simulink model "Quan"  (R2016a)
settings: Solver=VariableStepAuto  StartTime=0.0  StopTime=5000  FixedStep=0.1  RelTol=1e-3
settings Model: Creator=xin  LastModifiedBy=xin

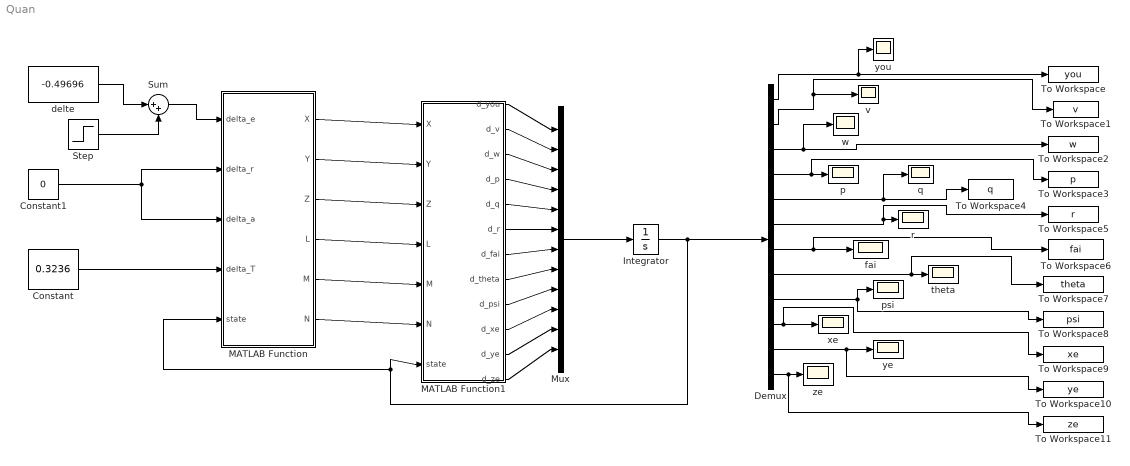
== system Quan ==
  Constant : Constant  Value=0.3236
  Constant1 : Constant  Value=0
  Demux : Demux  Outputs=12
  Integrator : Integrator  InitialCondition=[189.1684 0 17.7568 0 0 0 0 0.0936 0 0 0 0]
  MATLAB Function : MATLAB Function  TreatAsAtomicUnit=on
  MATLAB Function1 : MATLAB Function  TreatAsAtomicUnit=on
  Mux : Mux  Inputs=12
  Step : Step  Time=0  After=0.025  SampleTime=0
  Sum : Sum  Inputs=|++
  To Workspace : ToWorkspace  VariableName=you  SaveFormat=Timeseries  SampleTime=-1
  To Workspace1 : ToWorkspace  VariableName=v  SaveFormat=Timeseries  SampleTime=-1
  To Workspace10 : ToWorkspace  VariableName=ye  SaveFormat=Timeseries  SampleTime=-1
  To Workspace11 : ToWorkspace  VariableName=ze  SaveFormat=Timeseries  SampleTime=-1
  To Workspace2 : ToWorkspace  VariableName=w  SaveFormat=Timeseries  SampleTime=-1
  To Workspace3 : ToWorkspace  VariableName=p  SaveFormat=Timeseries  SampleTime=-1
  To Workspace4 : ToWorkspace  VariableName=q  SaveFormat=Timeseries  SampleTime=-1
  To Workspace5 : ToWorkspace  VariableName=r  SaveFormat=Timeseries  SampleTime=-1
  To Workspace6 : ToWorkspace  VariableName=fai  SaveFormat=Timeseries  SampleTime=-1
  To Workspace7 : ToWorkspace  VariableName=theta  SaveFormat=Timeseries  SampleTime=-1
  To Workspace8 : ToWorkspace  VariableName=psi  SaveFormat=Timeseries  SampleTime=-1
  To Workspace9 : ToWorkspace  VariableName=xe  SaveFormat=Timeseries  SampleTime=-1
  delte : Constant  Value=-0.49696
  fai : Scope
  p : Scope
  psi : Scope
  q : Scope
  r : Scope
  "theta " : Scope
  v : Scope
  w : Scope
  xe : Scope
  ye : Scope
  you : Scope
  "ze " : Scope
  wires:
  MATLAB Function/1(X) -> MATLAB Function1/1(X)
  MATLAB Function/2(Y) -> MATLAB Function1/2(Y)
  MATLAB Function/3(Z) -> MATLAB Function1/3(Z)
  MATLAB Function/4(L) -> MATLAB Function1/4(L)
  MATLAB Function/5(M) -> MATLAB Function1/5(M)
  MATLAB Function/6(N) -> MATLAB Function1/6(N)
  MATLAB Function1/1(d_you) -> Mux/1
  MATLAB Function1/2(d_v) -> Mux/2
  MATLAB Function1/3(d_w) -> Mux/3
  MATLAB Function1/4(d_p) -> Mux/4
  MATLAB Function1/5(d_q) -> Mux/5
  MATLAB Function1/6(d_r) -> Mux/6
  MATLAB Function1/7(d_fai) -> Mux/7
  MATLAB Function1/8(d_theta) -> Mux/8
  MATLAB Function1/10(d_xe) -> Mux/10
  MATLAB Function1/9(d_psi) -> Mux/9
  MATLAB Function1/11(d_ye) -> Mux/11
  MATLAB Function1/12(d_ze) -> Mux/12
  Integrator/1 -> MATLAB Function1/7(state), MATLAB Function/5(state), Demux/1
  Demux/1 -> you/1, To Workspace/1
  Demux/2 -> v/1, To Workspace1/1
  Demux/3 -> To Workspace2/1, w/1
  Demux/4 -> To Workspace3/1, p/1
  Demux/5 -> To Workspace4/1, q/1
  Demux/6 -> To Workspace5/1, r/1
  Demux/7 -> To Workspace6/1, fai/1
  Demux/8 -> To Workspace7/1, "theta "/1
  Demux/9 -> To Workspace8/1, psi/1
  Demux/10 -> To Workspace9/1, xe/1
  Demux/11 -> To Workspace10/1, ye/1
  Demux/12 -> To Workspace11/1, "ze "/1
  Constant/1 -> MATLAB Function/4(delta_T)
  Constant1/1 -> MATLAB Function/3(delta_a), MATLAB Function/2(delta_r)
  Mux/1 -> Integrator/1
  Sum/1 -> MATLAB Function/1(delta_e)
  delte/1 -> Sum/1
  Step/1 -> Sum/2

== matlab function Quan/MATLAB Function1 ==
  data: X input; d_you output; Y input; Z input; L input; M input; N input; state input; d_v output; d_w output; d_p output; d_q output; d_r output; d_fai output; d_theta output; d_psi output; d_xe output; d_ye output; d_ze output
function [d_you,d_v,d_w,d_p,d_q,d_r,d_fai,d_theta,d_psi,d_xe,d_ye,d_ze] = fcn(X, Y, Z, L, M, N, state)
%#codegen

you = state(1);
v = state(2);
w = state(3);
p = state(4);
q = state(5);
r = state(6);
fai = state(7);
theta = state(8);
psi = state(9);
ze = state(12);

H = 10000 - ze;
V = sqrt(you^2 + v^2 + w^2);

%--------在1000米出ze为0-------%
R = 6356766; g0 = 9.80665;

%-------飞机的惯性数据（国际单位制）---------%
m = 9298.643585;
Ix = 12874.8446;  Iy = 75673.6077;  Iz = 85552.0953;  Ixz = 1331.4130;  Isum=Ix*Iz-Ixz^2;
%xcg=0.3*c_;
%xcgr=0.35*c_;
c1=((Iy-Iz)*Iz-Ixz^2)/Isum;
c2=(Ix-Iy+Iz)*Ixz/Isum;
c3=Iz/Isum;
c4=Ixz/Isum;
c5=(Iz-Ix)/Iy;
c6=Ixz/Iy;
c7=1/Iy;
c8=(Ix*(Ix-Iy)+Ixz^2)/Isum;
c9=Ix/Isum;

%g = g0*(R/(R + H))^2;
g = 9.760531983853626;

%--------计算导数-------------%
%--------已知状态量 you; v; w; p; q; r; fai; theta; psi; -------------%
%--------  输入量 delta_T; delta_e; delta_a; delta_r; -------------%

d_you = X/m - g*sin(theta) - q*w + r*v;
d_v = Y/m + g*cos(theta)*sin(fai) - r*you + p*w;
d_w = Z/m+g*cos(theta)*cos(fai)-p*v+q*you;

d_p = (c1*r+c2*p)*q+c3*L+c4*N;
d_q = c5*p*r-c6*(p^2-q^2)+c7*M;
d_r = (c8*p-c2*r)*q+c4*L+c9*N;

d_fai = p+(q*sin(fai)+r*cos(fai))*tan(theta);
d_theta = q*cos(fai)-r*sin(fai);
d_psi = (q*sin(fai)+r*cos(fai))/cos(theta);

d_xe = you*cos(psi)*cos(theta) + v*(cos(psi)*sin(theta)*sin(fai)- sin(psi)*cos(fai)) + w*(cos(psi)*sin(theta)*cos(fai) + sin(psi)*sin(fai));
d_ye = you*sin(psi)*cos(theta) + v*(sin(psi)*sin(theta)*sin(fai) + cos(psi)*cos(fai)) + w*(sin(psi)*sin(theta)*cos(fai) - cos(psi)*sin(fai));
d_ze = -you*sin(theta) + v*cos(theta)*sin(fai) + w*cos(theta)*cos(fai);

%y = [d_you d_v d_w d_p d_q d_r d_fai d_theta d_psi d_xe d_ye d_ze H V];

== matlab function Quan/MATLAB Function ==
  data: delta_e input; X output; delta_r input; delta_a input; delta_T input; state input; Y output; Z output; L output; M output; N output
function [X, Y, Z, L, M, N] = fcn(delta_e, delta_r, delta_a, delta_T, state)

you = state(1);
v = state(2);
w = state(3);
p = state(4);
q = state(5);
r = state(6);
fai = state(7);
theta = state(8);
psi = state(9);
ze = state(12);

H = 10000 - ze;
V = sqrt(you^2 + v^2 + w^2);

%地球半径%
R = 6356766; 

%-------飞机的常数（国际单位制）---------%
c_= 3.4503;S = 27.8709;b = 9.144;r2d=57.29577951;

Vv = sqrt(you^2+v^2+w^2);

alpha = atan(w/you); 
beta = asin(v/Vv);

r2dalpha=r2d*alpha;
r2dbeta=r2d*beta;

%-------飞机的惯性数据（国际单位制）---------%
Ix = 12874.8446;  Iy = 75673.6077;  Iz = 85552.0953;  Ixz = 1331.4130;  Isum=Ix*Iz-Ixz^2;


%气动参数
given_Alpha = [-10 -5 0 5 10 15 20 25 30 35 40 45];
given_Elevator = [-24 -12 0	12 24];
given_Cz =[0.7700 0.2410 -0.1000 -0.4160 -0.7310 -1.0530 -1.3660 -1.6460 -1.9170 -2.1200 -2.2480 -2.2290];
given_Cx = [-0.099	-0.048	-0.022	-0.04	-0.083
    -0.081	-0.038	-0.02	-0.038	-0.073
    -0.081	-0.04	-0.021	-0.039	-0.076
    -0.063	-0.021	-0.004	-0.025	-0.072
    -0.025	 0.016	 0.032	 0.006	-0.046
    0.044	 0.083	 0.094	 0.062	 0.012
    0.097	 0.127	 0.128	 0.087	 0.024
    0.113	 0.137	 0.13	 0.085	 0.025
    0.145	 0.162	 0.154	 0.1	 0.043
    0.167	 0.177	 0.161	 0.11	 0.053
    0.174	 0.179	 0.155	 0.104	 0.047
    0.166	 0.167	 0.138	 0.091	 0.04];
given_Cm = [0.205	 0.081	-0.046	-0.174	-0.259
    0.168	 0.077	-0.02	-0.145	-0.202
    0.186	 0.107	-0.009	-0.121	-0.184
    0.196	 0.11	-0.005	-0.127	-0.193
    0.213	 0.11	-0.006	-0.129	-0.199
    0.251	 0.141	 0.01	-0.102	-0.15
    0.245	 0.127	 0.006	-0.097	-0.16
    0.238	 0.119	-0.001	-0.113	-0.167
    0.252	 0.133	 0.014	-0.087	-0.104
    0.231  0.108	 0	    -0.084	-0.076
    0.198	 0.081	-0.013	-0.069	-0.041
    0.192	 0.093	 0.032	-0.006	-0.005];
given_Cl = [0	-0.001	-0.003	-0.001	 0	     0.07	 0.009
    0	-0.004	-0.009	-0.01	-0.01	-0.01	-0.011
    0	-0.008	-0.017	-0.02	-0.022	-0.023	-0.023
    0	-0.012	-0.024	-0.03	-0.034	-0.034	-0.037
    0	-0.016	-0.03	-0.039	-0.047	-0.049	-0.05
    0	-0.019	-0.034	-0.044	-0.046	-0.046	-0.047
    0	-0.02	-0.04	-0.05	-0.059	-0.068	-0.074
    0	-0.02	-0.037	-0.049	-0.061	-0.071	-0.079
    0	-0.015	-0.016	-0.023	-0.033	-0.06	-0.091
    0	-0.008	-0.002	-0.006	-0.036	-0.058	-0.076
    0	-0.013	-0.1	-0.014	-0.035	-0.062	-0.077
    0	-0.015	-0.19	-0.027	-0.035	-0.059	-0.076];
given_Cn = [0	0.018	0.038	0.056	0.064	0.074	0.079
    0	0.019	0.042	0.057	0.077	0.086	0.09
    0	0.018	0.042	0.059	0.076	0.093	0.106
    0	0.019	0.042	0.058	0.074	0.089	0.106
    0	0.019	0.043	0.058	0.073	0.08	0.096
    0	0.018	0.039	0.053	0.057	0.062	0.08
    0	0.013	0.03	0.032	0.029	0.049	0.068
    0	0.007	0.017	0.012	0.007	0.022	0.03
    0	0.004	0.004	0.002	0.012	0.028	0.064
    0  -0.014  -0.035  -0.046  -0.034  -0.012	0.015
    0  -0.017  -0.047  -0.071  -0.065  -0.002	0.011
    0  -0.033  -0.057  -0.073  -0.041  -0.013  -0.001];
given_Cl_delta_a = [-0.041	-0.041	-0.042	-0.04	-0.043	-0.044	-0.043
    -0.052	-0.053	-0.053	-0.052	-0.049	-0.048	-0.049
    -0.053	-0.053	-0.052	-0.051	-0.048	-0.048	-0.047
    -0.056	-0.053	-0.051	-0.052	-0.049	-0.047	-0.045
    -0.05	-0.05	-0.049	-0.048	-0.043	-0.042	-0.042
    -0.056	-0.051	-0.049	-0.048	-0.042	-0.041	-0.037
    -0.082	-0.066	-0.043	-0.042	-0.042	-0.02	-0.003
    -0.059	-0.043	-0.035	-0.037	-0.036	-0.028	-0.013
    -0.042	-0.038	-0.026	-0.031	-0.025	-0.013	-0.01
    -0.038	-0.027	-0.016	-0.026	-0.021	-0.014	-0.003
    -0.027	-0.023	-0.018	-0.017	-0.016	-0.011	-0.007
    -0.017	-0.016	-0.014	-0.012	-0.011	-0.01	-0.008];
given_Cl_delta_r = [0.005	0.007	0.013	0.018	0.015	0.021	0.023
    0.017	0.016	0.013	0.015	0.014	0.011	0.01
    0.014	0.014	0.011	0.015	0.013	0.01	0.011
    0.01    0.014	0.012	0.014	0.013	0.011	0.011
    -0.005	0.013	0.011	0.014	0.012	0.01	0.011
    0.009	0.009	0.009	0.014	0.011	0.009	0.01
    0.019	0.012	0.008	0.014	0.011	0.008	0.008
    0.005	0.005	0.005	0.015	0.01	0.01	0.01
    0	    0	   -0.002	0.013	0.008	0.006	0.006
    -0.005	0.004	0.005	0.011	0.008	0.005	0.014
    -0.011	0.009	0.003	0.006	0.007	0	    0.02
    0.008	0.007	0.005	0.001	0.003	0.001	0    ];
given_Cn_delta_a = [0.001	 0.002	-0.006	-0.011	-0.015	-0.024	-0.022
    -0.027	-0.014	-0.008	-0.011	-0.015	-0.01	 0.002
    -0.017	-0.016	-0.006	-0.01	-0.014	-0.004	-0.003
    -0.013	-0.016	-0.006	-0.009	-0.012	-0.002	-0.005
    -0.012	-0.014	-0.005	-0.008	-0.011	-0.001	-0.003
    -0.016	-0.019	-0.008	-0.006	-0.008	 0.003	-0.001
    0.001	-0.021	-0.005	 0	    -0.002	 0.014	-0.009
    0.017	 0.002	 0.007	 0.004	 0.002	 0.006	-0.009
    0.011	 0.012	 0.004	 0.007	 0.006	-0.001	-0.001
    0.017	 0.015	 0.007	 0.1	 0.012	 0.004	 0.003
    0.008	 0.015	 0.006	 0.004	 0.011	 0.004	-0.002
    0.016	 0.011	 0.006	 0.1	 0.011	 0.006	 0.001];
given_Cn_delta_r = [-0.018	-0.028	-0.037	-0.048	-0.043	-0.052	-0.062
    -0.052	-0.051	-0.041	-0.045	-0.044	-0.034	-0.034
    -0.052	-0.043	-0.038	-0.045	-0.041	-0.036	-0.027
    -0.052	-0.046	-0.04	-0.045	-0.041	-0.036	-0.028
    -0.054	-0.045	-0.04	-0.044	-0.04	-0.035	-0.027
    -0.049	-0.049	-0.038	-0.045	-0.038	-0.028	-0.027
    -0.059	-0.057	-0.037	-0.047	-0.034	-0.024	-0.023
    -0.051	-0.052	-0.03	-0.048	-0.035	-0.023	-0.023
    -0.03	-0.03	-0.027	-0.049	-0.035	-0.02	-0.019
    -0.037	-0.033	-0.024	-0.045	-0.029	-0.016	-0.009
    -0.026	-0.03	-0.019	-0.033	-0.022	-0.01	-0.025
    -0.013	-0.008	-0.013	-0.016	-0.009	-0.014	-0.01];
given_throtte_000=[1060	  670	 880	 1140	1500	1860
    635	  425	 690	 1010	1330	1700
    60	  25	 345	 755	1130	1525
    -1020	 -710	-300	 350	910	    1360
    -2700	 -1900	-1300	-247	600	    1100
    -3600	 -1400	-595	-342   -200	    700];
given_throtte_077=[12680	9150	6200	3950	2450	1400
    12680	9150	6313	4040	2470	1400
    12610	9312	6610	4290	2600	1560
    12640	9839	7090	4660	2840	1660
    12390	10176	7750	5320	3250	1930
    11680	9848	8050	6100	3800	2310];
given_throtte_100=[20000	15000	10800	7000	4000	2500
    21420	15700	11225	7323	4435	2600
    22700	16860	12250	8154	5000	2835
    24240	18910	13760	9285	5700	3215
    26070	21075	15975	11115	6860	3950
    28886	23319	18300	13484	8642	5057];

given_Cxq = [-0.267 -0.11 0.308 1.34 2.08 2.91 2.76 2.05 1.5 1.49 1.83 1.21];
given_Cyr = [0.882 0.852 0.876 0.958 0.962 0.974 0.819 0.483 0.59 1.21 -0.493 -1.04];
given_Cyp = [-0.108 -0.108 -0.188 0.11 0.258 0.226 -0.344 0.362 0.611 0.529 0.298 -2.27];
given_Czq = [-8.8 -25.8 -28.9 -31.4 -31.2 -30.7 -27.7 -28.2 -29 -29.8 -38.3 -35.3];
given_Clr = [-0.126 -0.126 0.063 0.113 0.208 0.23 0.319 0.437 0.68 0.1 0.447 -0.33];
given_Clp = [-0.36 -0.359 -0.443 -0.42 -0.383 -0.375 -0.329 -0.294 -0.23 -0.21 -0.12 -0.1];
given_Cmq = [-7.21 -0.54 -5.23 -5.26 -6.11 -6.64 -5.69 -6 -6.2 -6.4 -6.6 -6];
given_Cnr = [-0.38 -0.363 -0.378 -0.386 -0.37 -0.453 -0.55 -0.582 -0.595 -0.637 -1.02 -0.804];
given_Cnp = [0.061 0.052 0.052 -0.012 -0.013 -0.024 0.05 0.15 0.13 0.158 0.24 0.15];

given_delta_beta = [-30	-20	-10	0 10 20	30];
given_beta = [0	5 10 15	20	25	30];

%%---------发动机推力插值，（英美单位制）-------------%%
given_height=[0	10000 20000	30000 40000	50000];
given_mah=[0 0.2 0.4 0.6 0.8 1]';


%海平面大气密度%
rou0 = 1.225;

%大气分层的几个分层点%
h1 = 11019.1;
h2 = 20063.1;


%----------计算温度，大气密度-----------%
h_p = R*H/((R + H)*1000);
if H>=0 && H<=h1;
    WW = 1-h_p/44.3308;
    T = 288.15*WW;
    rou = rou0*WW^4.2559;
elseif H>=h1 && H<=h2;
    WW = exp((14.9647-h_p)/6.3416);
    T = 216.650;
    rou = 1.5898*10^(-1)*rou0*WW;
else
    WW = 0;
    T = 0*WW;
    rou = 0;
end

%-----------计算声速---------------%
a = 20.0468*T^0.5;
Mah = V/a;

%-------------计算气动导数-------------------%
Cx_q = interp1(given_Alpha,given_Cxq,r2dalpha,'spline');
Cy_r = interp1(given_Alpha,given_Cyr,r2dalpha,'spline');
Cy_p = interp1(given_Alpha,given_Cyp,r2dalpha,'spline');
Cz_q = interp1(given_Alpha,given_Czq,r2dalpha,'spline');
Cl_r = interp1(given_Alpha,given_Clr,r2dalpha,'spline');
Cl_p = interp1(given_Alpha,given_Clp,r2dalpha,'spline');
Cm_q = interp1(given_Alpha,given_Cmq,r2dalpha,'spline');
Cn_r = interp1(given_Alpha,given_Cnr,r2dalpha,'spline');
Cn_p = interp1(given_Alpha,given_Cnp,r2dalpha,'spline');

Interp_throtte_000=interp2(given_height,given_mah,given_throtte_000,H/0.3048,Mah,'spline')*(14.5939*0.3048);
Interp_throtte_077=interp2(given_height,given_mah,given_throtte_077,H/0.3048,Mah,'spline')*(14.5939*0.3048);
Interp_throtte_100=interp2(given_height,given_mah,given_throtte_100,H/0.3048,Mah,'spline')*(14.5939*0.3048);
matrix_interp=[Interp_throtte_000 Interp_throtte_077 Interp_throtte_100];
throtte_value=[0 0.77 1];
X_thrust = interp1(throtte_value,matrix_interp,delta_T);

Cx=interp2(given_Elevator,given_Alpha,given_Cx,delta_e,r2dalpha,'spline')+Cx_q*q*c_/(2*V);
Cy=-0.02*r2dbeta+0.021*(delta_a/20)+0.086*(delta_r/30)+b/(2*V)*(Cy_p*p+Cy_r*r);
Cz=interp1(given_Alpha,given_Cz,r2dalpha,'spline')*(1-beta^2)-0.19*(delta_e/25.0)+Cz_q*q*c_/(2*V);

Cl_delta_a=interp2(given_delta_beta,given_Alpha,given_Cl_delta_a,r2dbeta,r2dalpha,'spline');
Cl_delta_r=interp2(given_delta_beta,given_Alpha,given_Cl_delta_r,r2dbeta,r2dalpha,'spline');
Cl=sign(r2dbeta)*interp2(given_beta,given_Alpha,given_Cl,abs(r2dbeta),r2dalpha,'spline')...
    +Cl_delta_a*delta_a+Cl_delta_r*delta_r+b/(2*V)*(Cl_p*p+Cl_r*r);

Cm=interp2(given_Elevator,given_Alpha,given_Cm,delta_e,r2dalpha,'spline')+Cm_q*q*c_/(2*V);%;

Cn_delta_a=interp2(given_delta_beta,given_Alpha,given_Cn_delta_a,r2dbeta,r2dalpha,'spline');
Cn_delta_r=interp2(given_delta_beta,given_Alpha,given_Cn_delta_r,r2dbeta,r2dalpha,'spline');
Cn=sign(r2dbeta)*interp2(given_beta,given_Alpha,given_Cn,abs(r2dbeta),r2dalpha,'spline')...
    +Cn_delta_a*delta_a+Cn_delta_r*delta_r+b/(2*V)*(Cn_r*r+Cn_p*p);%;


%-------计算力和力矩------------%
X = X_thrust+0.5*rou*V^2*S*Cx;
Y = 0.5*rou*V^2*S*Cy;
Z = 0.5*rou*V^2*S*Cz;
L = 0.5*rou*V^2*S*b*Cl;
M = 0.5*rou*V^2*S*c_*Cm;
N = 0.5*rou*V^2*S*b*Cn;

%y = [X, Y, Z, L, M, N];
